simulink model "xtrack"  (Simulink 7.9)
settings: Solver=ode45  StartTime=0.0  StopTime=6.0  RelTol=1e-3
values from neighbouring files (symbols this model uses):
  A = 0.002    [params.m]
  v = 100    [params.m]
libraries: simulink x1
settings Model: Creator=dave  LastModifiedBy=dave

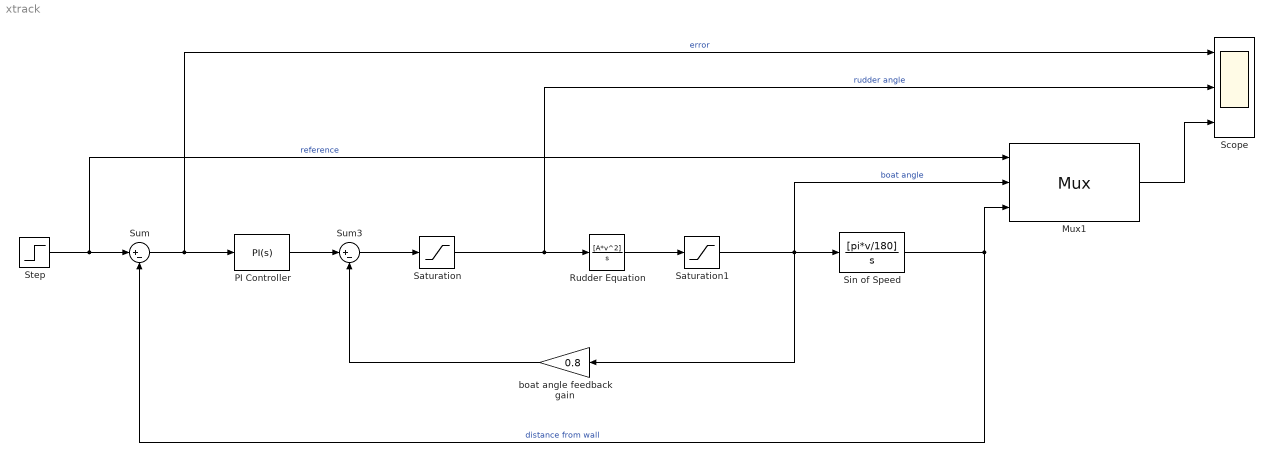
== system xtrack ==
  Mux1 : Mux  Inputs=3
      settings: DisplayOption=signals
  PI Controller : simulink/Continuous/PID Controller  Controller=PI  TimeDomain=Continuous-time  SampleTime=1  IntegratorMethod=Forward Euler  FilterMethod=Forward Euler  Form=Parallel  P=1  I=0  D=0  N=7.02962681019428  InitialConditionSource=internal  InitialConditionForIntegrator=0  InitialConditionForFilter=0  ExternalReset=none  LimitOutput=off  UpperSaturationLimit=inf  LowerSaturationLimit=-inf  LinearizeAsGain=off  AntiWindupMode=none  Kb=1  TrackingMode=off  Kt=1  PParamMin=[]  PParamMax=[]  IParamMin=[]  IParamMax=[]  DParamMin=[]  DParamMax=[]  NParamMin=[]  NParamMax=[]  KbParamMin=[]  KbParamMax=[]  KtParamMin=[]  KtParamMax=[]  POutMin=[]  POutMax=[]  IOutMin=[]  IOutMax=[]  DOutMin=[]  DOutMax=[]  NOutMin=[]  NOutMax=[]  KbOutMin=[]  KbOutMax=[]  KtOutMin=[]  KtOutMax=[]  IntegratorOutMin=[]  IntegratorOutMax=[]  FilterOutMin=[]  FilterOutMax=[]  SumOutMin=[]  SumOutMax=[]  SumI1OutMin=[]  SumI1OutMax=[]  SumI2OutMin=[]  SumI2OutMax=[]  SumI3OutMin=[]  SumI3OutMax=[]  SumDOutMin=[]  SumDOutMax=[]  SaturationOutMin=[]  SaturationOutMax=[]  IntegratorContinuousStateAttributes=''  IntegratorStateMustResolveToSignalObject=off  IntegratorRTWStateStorageClass=Auto  FilterContinuousStateAttributes=''  FilterStateMustResolveToSignalObject=off  FilterRTWStateStorageClass=Auto
  Rudder Equation : TransferFcn  Numerator=[A*v^2]  Denominator=[1 0]
  Saturation : Saturate  UpperLimit=25  LowerLimit=-25
  Saturation1 : Saturate  UpperLimit=100  LowerLimit=-100
  Scope : Scope  NumInputPorts=3
      settings: ShowLegends=on  TimeRange=6  YMin=-50~-30~-40  YMax=50~30~100
  Sin of Speed : TransferFcn  Numerator=[pi*v/180]  Denominator=[1 0]
  Step : Step  After=40  SampleTime=0
  Sum : Sum  Inputs=|+-
  Sum3 : Sum  Inputs=|+-
  boat angle feedback gain : Gain  Gain=0.8
  wires:
  Sum/1 -> PI Controller/1, Scope/1  "error"
  Step/1 -> Sum/1, Mux1/1  "reference"
  Mux1/1 -> Scope/3
  Sin of Speed/1 -> Sum/2, Mux1/3  "distance from wall"
  PI Controller/1 -> Sum3/1
  Sum3/1 -> Saturation/1
  boat angle feedback gain/1 -> Sum3/2
  Rudder Equation/1 -> Saturation1/1
  Saturation1/1 -> Sin of Speed/1, boat angle feedback gain/1, Mux1/2  "boat angle"
  Saturation/1 -> Rudder Equation/1, Scope/2  "rudder angle"
